simulink model "sim_lec15_eul"  (R2016b)
settings: Solver=VariableStepAuto  StartTime=0.0  StopTime=60.0  RelTol=1e-3
undefined symbols (not defined in the file or in its folder): sim_params
libraries: aerolibutil x2, vrlib x1, aerolibtransform2 x1
settings Model: Creator=taylorreynolds  LastModifiedBy=Taylor

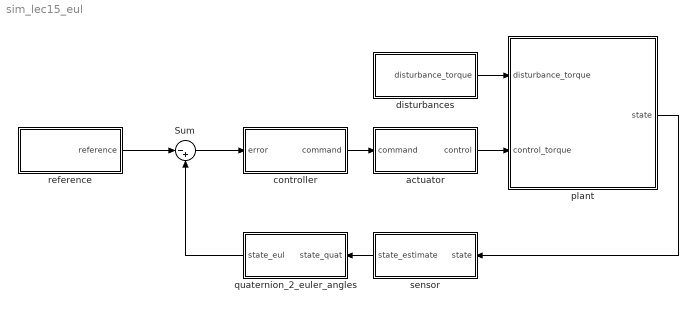
== system sim_lec15_eul ==
  Sum : Sum  Inputs=|-+
  actuator : Subsystem
  controller : Subsystem
  disturbances : Subsystem
  plant : Subsystem
  quaternion_2_euler_angles : Subsystem
  reference : Subsystem
  sensor : Subsystem
  wires:
  actuator/1(control) -> plant/2(control_torque)
  disturbances/1(disturbance_torque) -> plant/1(disturbance_torque)
  plant/1(state) -> sensor/1(state)
  controller/1(command) -> actuator/1(command)
  Sum/1 -> controller/1(error)
  quaternion_2_euler_angles/1(state_eul) -> Sum/2
  reference/1(reference) -> Sum/1
  sensor/1(state_estimate) -> quaternion_2_euler_angles/1(state_quat)

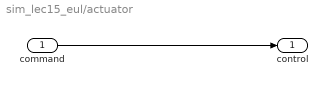
== system sim_lec15_eul/actuator ==
  command : Inport
  control : Outport
  wires:
  command/1 -> control/1

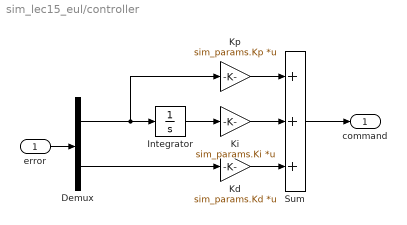
== system sim_lec15_eul/controller ==
  error : Inport
  Demux : Demux  Outputs=[3 3]
  Integrator : Integrator
  Kd : Gain  Gain=sim_params.Kd  Multiplication=Matrix(K*u)
  Ki : Gain  Gain=sim_params.Ki  Multiplication=Matrix(K*u)
  Kp : Gain  Gain=sim_params.Kp  Multiplication=Matrix(K*u)
  Sum : Sum  Inputs=+++
  command : Outport
  wires:
  error/1 -> Demux/1
  Sum/1 -> command/1
  Integrator/1 -> Ki/1
  Demux/2 -> Kd/1
  Kd/1 -> Sum/3
  Ki/1 -> Sum/2
  Kp/1 -> Sum/1
  Demux/1 -> Kp/1, Integrator/1

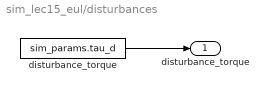
== system sim_lec15_eul/disturbances ==
  "disturbance_torque " : Constant  Value=sim_params.tau_d
  disturbance_torque : Outport
  wires:
  "disturbance_torque "/1 -> disturbance_torque/1

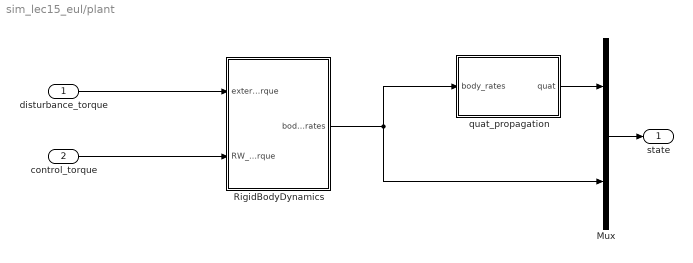
== system sim_lec15_eul/plant ==
  disturbance_torque : Inport
  control_torque : Inport  Port=2
  Mux : Mux  Inputs=[4 3]
  RigidBodyDynamics : Subsystem
  quat_propagation : Subsystem
  state : Outport
  wires:
  RigidBodyDynamics/1(body_rates) -> Mux/2, quat_propagation/1(body_rates)
  disturbance_torque/1 -> RigidBodyDynamics/1(external_torque)
  control_torque/1 -> RigidBodyDynamics/2(RW_torque)
  quat_propagation/1(quat) -> Mux/1
  Mux/1 -> state/1

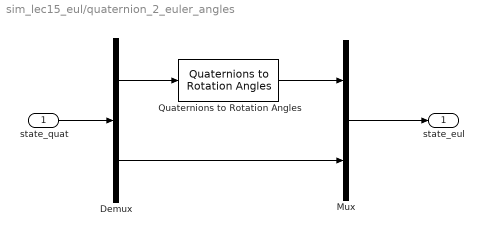
== system sim_lec15_eul/quaternion_2_euler_angles ==
  state_quat : Inport
  Demux : Demux  Outputs=[4 3]
  Mux : Mux  Inputs=[3 3]
  Quaternions to Rotation Angles : aerolibtransform2/Quaternions to Rotation Angles  rotationOrder=XYZ
  state_eul : Outport
  wires:
  state_quat/1 -> Demux/1
  Demux/1 -> Quaternions to Rotation Angles/1
  Demux/2 -> Mux/2
  Mux/1 -> state_eul/1
  Quaternions to Rotation Angles/1 -> Mux/1

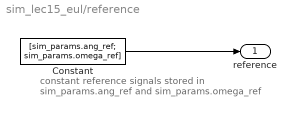
== system sim_lec15_eul/reference ==
  note: constant reference signals stored in sim_params.ang_ref and
      | sim_params.omega_ref
  Constant : Constant  Value=[sim_params.ang_ref; sim_params.omega_ref]
  reference : Outport
  wires:
  Constant/1 -> reference/1

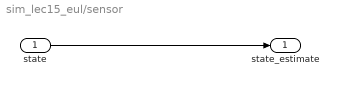
== system sim_lec15_eul/sensor ==
  state : Inport
  state_estimate : Outport
  wires:
  state/1 -> state_estimate/1

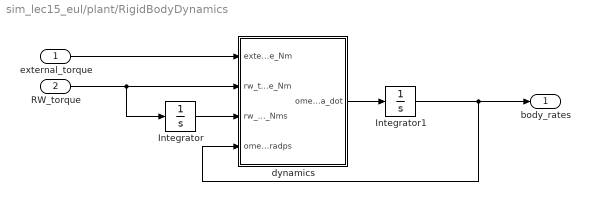
== system sim_lec15_eul/plant/RigidBodyDynamics ==
  external_torque : Inport
  RW_torque : Inport  Port=2
  Integrator : Integrator  InitialCondition=sim_params.ic.rw_momentum
  Integrator1 : Integrator  InitialCondition=sim_params.ic.omega_radps
  dynamics : Subsystem
  body_rates : Outport
  wires:
  dynamics/1(omega_dot) -> Integrator1/1
  external_torque/1 -> dynamics/1(external_torque_Nm)
  Integrator1/1 -> dynamics/4(omega_radps), body_rates/1
  Integrator/1 -> dynamics/3(rw_momentum_Nms)
  RW_torque/1 -> Integrator/1, dynamics/2(rw_torque_Nm)

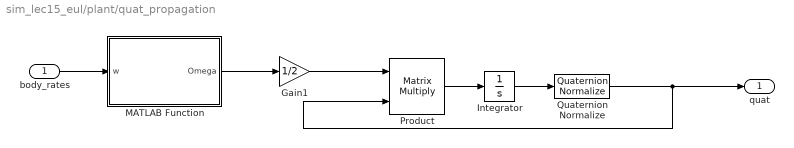
== system sim_lec15_eul/plant/quat_propagation ==
  body_rates : Inport
  Gain1 : Gain  Gain=1/2
  Integrator : Integrator  InitialCondition=sim_params.ic.quaternion
  MATLAB Function : MATLAB Function  TreatAsAtomicUnit=on
  Product : Product  Multiplication=Matrix(*)  RndMeth=Zero
  Quaternion Normalize : aerolibutil/Quaternion Normalize
  quat : Outport
  wires:
  MATLAB Function/1(Omega) -> Gain1/1
  body_rates/1 -> MATLAB Function/1(w)
  Quaternion Normalize/1 -> Product/2, quat/1
  Gain1/1 -> Product/1
  Integrator/1 -> Quaternion Normalize/1
  Product/1 -> Integrator/1

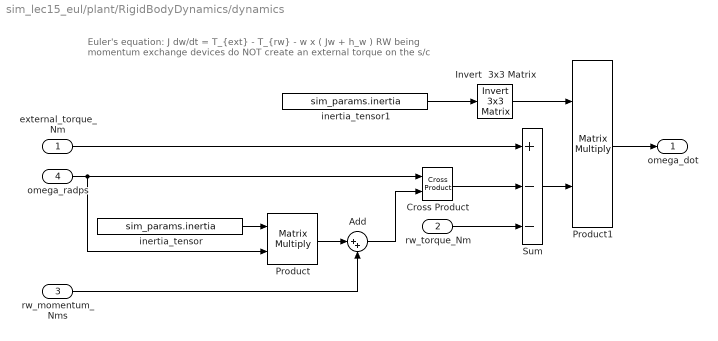
== system sim_lec15_eul/plant/RigidBodyDynamics/dynamics ==
  note: Euler's equation: J dw/dt = T_{ext} - T_{rw} - w x ( Jw + h_w )
      |
      | RW being momentum exchange devices do NOT create
      | an external torque on the s/c
  external_torque_Nm : Inport
  rw_torque_Nm : Inport  Port=2
  rw_momentum_Nms : Inport  Port=3
  omega_radps : Inport  Port=4
  Add : Sum  Inputs=|++
  Cross Product : vrlib/Utilities/Cross Product
  Invert  3x3 Matrix : aerolibutil/Invert  3x3 Matrix
  Product : Product  Multiplication=Matrix(*)  RndMeth=Zero
  Product1 : Product  Multiplication=Matrix(*)  RndMeth=Zero
  Sum : Sum  Inputs=+--
  inertia_tensor : Constant  Value=sim_params.inertia
  inertia_tensor1 : Constant  Value=sim_params.inertia
  omega_dot : Outport
  wires:
  external_torque_Nm/1 -> Sum/1
  omega_radps/1 -> Product/2, Cross Product/1
  inertia_tensor/1 -> Product/1
  Sum/1 -> Product1/2
  Product1/1 -> omega_dot/1
  Invert  3x3 Matrix/1 -> Product1/1
  inertia_tensor1/1 -> Invert  3x3 Matrix/1
  Cross Product/1 -> Sum/2
  Product/1 -> Add/1
  rw_momentum_Nms/1 -> Add/2
  Add/1 -> Cross Product/2
  rw_torque_Nm/1 -> Sum/3

== matlab function sim_lec15_eul/plant/quat_propagation/MATLAB Function ==
  data: w input; Omega output
function Omega = skew_sym(w)
%#codegen

    w_skew = ...
        [0 w(3) -w(2);
        -w(3) 0 w(1);
        w(2) -w(1) 0];

% Omega = [ w_skew w;
%     -w' 0.0 ];

Omega = [ 0.0 -w';
          w    w_skew ];
        
end
